simulink library "lib_controls"  (Simulink 7.9)
settings: Solver=ode45  SolverMode=SingleTasking  StartTime=0.0  StopTime=10.0  RelTol=1e-3
undefined symbols (not defined in the file or in its folder): amb_tmp, cs_charge_deplete_bool, cs_charge_pwr, cs_charge_trq, cs_clt_tmp, cs_decel_fc_off, cs_decel_regen_threshold, cs_dl_assist_trq_threshold, cs_dl_regen_trq_threshold, cs_electric_decel_spd, cs_electric_launch_spd, cs_electric_launch_spd_hi, cs_electric_launch_spd_lo, cs_eng_min_spd, cs_eng_on_soc, cs_fc_init_state, cs_fc_max_pwr_frac, cs_fc_min_pwr_frac, cs_fc_on, cs_fc_pwr_opt, cs_fc_spd_opt, cs_fuzzy_fuel_mode, cs_hi_soc, cs_hi_trq_frac, cs_lo_soc, cs_lo_trq_frac, cs_max_gc_spd, cs_max_pwr, cs_max_pwr_fall_rate, cs_max_pwr_rise_rate, cs_mc_assist_max_frac, cs_mc_assist_min_frac, cs_mc_assist_slope, cs_mc_regen_max_frac, cs_mc_regen_min_frac, cs_mc_regen_slope, cs_mean_eff, cs_mean_eff_bool, cs_min_gc_spd, cs_min_off_time, cs_min_pwr, cs_min_trq_frac, cs_mph_avg_time, cs_off_trq_frac, cs_plot_output, cs_pwr, cs_regen_avg_time, cs_scale_factor, cs_shutoff, cs_soc_range, cs_spd, cs_target_soc, cs_trq_to_soc_factor, cvt_locus_pwr, cvt_locus_spd, cyc_mph, enable_sim_stop_distance, enable_sim_stop_max_spd, enable_sim_stop_speed, enable_sim_stop_time ... (+110)
libraries: lib_controls x124, simulink3 x13, simulink x5, lib_etc x1
(part 15 of 17)

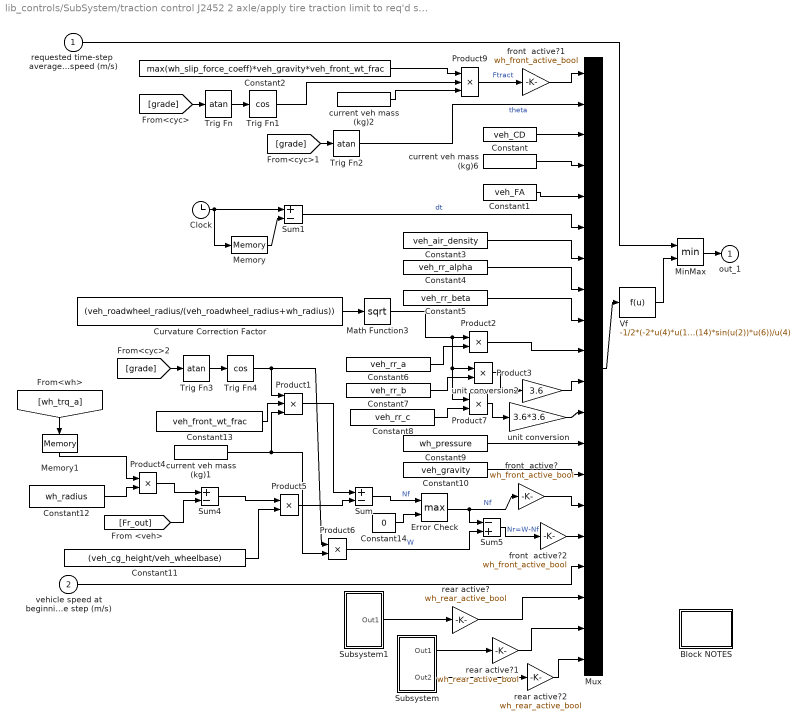
== system lib_controls/SubSystem/traction control J2452 2 axle/apply tire traction limit to req'd speed (m/s) ==
  "requested time-step  average vehicle speed (m/s) " : Inport
  vehicle speed at beginning of time step (m/s) : Inport  Port=2
  Block NOTES : Subsystem
      mask Display: disp('Block\nNOTES')
  Clock : Clock
  Constant : Constant  Value=veh_CD
  Constant1 : Constant  Value=veh_FA
  Constant10 : Constant  Value=veh_gravity
  Constant11 : Constant  Value=(veh_cg_height/veh_wheelbase)
  Constant12 : Constant  Value=wh_radius
  Constant13 : Constant  Value=veh_front_wt_frac
  Constant14 : Constant  Value=0
  Constant2 : Constant  Value=max(wh_slip_force_coeff)*veh_gravity*veh_front_wt_frac
  Constant3 : Constant  Value=veh_air_density
  Constant4 : Constant  Value=veh_rr_alpha
  Constant5 : Constant  Value=veh_rr_beta
  Constant6 : Constant  Value=veh_rr_a
  Constant7 : Constant  Value=veh_rr_b
  Constant8 : Constant  Value=veh_rr_c
  Constant9 : Constant  Value=wh_pressure
  Curvature Correction Factor : Constant  Value=(veh_roadwheel_radius/(veh_roadwheel_radius+wh_radius))  VectorParams1D=off
  Error Check : MinMax  Function=max  Inputs=2  SaturateOnIntegerOverflow=on  InputSameDT=on
  Math Function3 : Math  Operator=sqrt  SaturateOnIntegerOverflow=on
  Memory : Memory  X0=-0.1
  Memory1 : Memory  X0=-0.1
  MinMax : MinMax  Inputs=2  SaturateOnIntegerOverflow=on  InputSameDT=on
  Mux : Mux  Inputs=20
  Product1 : Product  Inputs=3  SaturateOnIntegerOverflow=on  RndMeth=Zero  InputSameDT=on  OutDataTypeStr=Inherit: Same as first input
  Product{2..7} (6 alike) : Product  SaturateOnIntegerOverflow=on  RndMeth=Zero  InputSameDT=on  OutDataTypeStr=Inherit: Same as first input
  Product9 : Product  Inputs=3  SaturateOnIntegerOverflow=on  RndMeth=Zero  InputSameDT=on  OutDataTypeStr=Inherit: Same as first input
  Subsystem : Subsystem
  Subsystem1 : Subsystem
  Sum : Sum  Inputs=+-  SaturateOnIntegerOverflow=on  InputSameDT=on  OutDataTypeStr=Inherit: Same as first input
  Sum1 : Sum  Inputs=+-  SaturateOnIntegerOverflow=on  InputSameDT=on  OutDataTypeStr=Inherit: Same as first input
  Sum4 : Sum  Inputs=+-  SaturateOnIntegerOverflow=on  InputSameDT=on  OutDataTypeStr=Inherit: Same as first input
  Sum5 : Sum  Inputs=-+  SaturateOnIntegerOverflow=on  InputSameDT=on  OutDataTypeStr=Inherit: Same as first input
  Trig Fn : Trigonometry  Operator=atan
  Trig Fn1 : Trigonometry  Operator=cos
  Trig Fn2 : Trigonometry  Operator=atan
  Trig Fn3 : Trigonometry  Operator=atan
  Trig Fn4 : Trigonometry  Operator=cos
  Vf : Fcn  Expr=-1/2*(-2*u(4)*u(17)-2*u(1)*u(6)-2*u(18)*u(6)+4*u(13)^u(8)*u(6)*(1/2*u(15))^u(9)*u(10)+4*u(13)^u(8)*u(6)*(1/2*u(19))^u(9)*u(10)+4*u(13)^u(8)*u(6)*(1/2*u(15))^u(9)*u(11)*u(17)+4*u(13)^u(8)*u(6)*(1/2*u(19))^u(9)*u(11)*u(17)+4*u(13)^u(8)*u(6)*(1/2*u(15))^u(9)*u(12)*u(17)^2+4*u(13)^u(8)*u(6)*(1/2*u(19))^u(9)*u(12)*u(17)^2+4*u(13)^u(8)*u(6)*(1/2*u(16))^u(9)*u(10)+4*u(13)^u(8)*u(6)*(1/2*u(20))^u(9)*u(10)+4*u(13)^u(8)*u(6)*(1/2*u(16))^u(9)*u(11)*u(17)+4*u(13)^u(8)*u(6)*(1/2*u(20))^u(9)*u(11)*u(17)+4*u(13)^u(8)*u(6)*(1/2*u(16))^u(9)*u(12)*u(17)^2+4*u(13)^u(8)*u(6)*(1/2*u(20))^u(9)*u(12)*u(17)^2+u(7)*u(3)*u(5)*u(17)^2*u(6)+2*u(4)*u(14)*sin(u(2))*u(6))/u(4)
  current veh mass (kg)1 : lib_controls/SubSystem/current veh mass (kg)
      settings: RTWFcnNameOpts=Auto  RTWFileNameOpts=Auto
  current veh mass (kg)2 : lib_controls/SubSystem/current veh mass (kg)
      settings: RTWFcnNameOpts=Auto  RTWFileNameOpts=Auto
  current veh mass (kg)6 : lib_controls/SubSystem/current veh mass (kg)
      settings: RTWFcnNameOpts=Auto  RTWFileNameOpts=Auto
  front  active? : Gain  Gain=wh_front_active_bool  SaturateOnIntegerOverflow=on  OutDataTypeStr=Inherit: Same as input  ParamDataTypeStr=Inherit: Same as input
  front  active?1 : Gain  Gain=wh_front_active_bool  SaturateOnIntegerOverflow=on  OutDataTypeStr=Inherit: Same as input  ParamDataTypeStr=Inherit: Same as input
  front  active?2 : Gain  Gain=wh_front_active_bool  SaturateOnIntegerOverflow=on  OutDataTypeStr=Inherit: Same as input  ParamDataTypeStr=Inherit: Same as input
  rear active? : Gain  Gain=wh_rear_active_bool  SaturateOnIntegerOverflow=on  OutDataTypeStr=Inherit: Same as input  ParamDataTypeStr=Inherit: Same as input
  rear active?1 : Gain  Gain=wh_rear_active_bool  SaturateOnIntegerOverflow=on  OutDataTypeStr=Inherit: Same as input  ParamDataTypeStr=Inherit: Same as input
  rear active?2 : Gain  Gain=wh_rear_active_bool  SaturateOnIntegerOverflow=on  OutDataTypeStr=Inherit: Same as input  ParamDataTypeStr=Inherit: Same as input
  unit conversion : Gain  Gain=3.6*3.6  SaturateOnIntegerOverflow=on  OutDataTypeStr=Inherit: Same as input  ParamDataTypeStr=Inherit: Same as input
  unit conversion2 : Gain  Gain=3.6  SaturateOnIntegerOverflow=on  OutDataTypeStr=Inherit: Same as input  ParamDataTypeStr=Inherit: Same as input
  out_1 : Outport  InitialOutput=0
  wires:
  Product7/1 -> unit conversion/1
  Constant8/1 -> Product7/2
  Product3/1 -> unit conversion2/1
  Constant7/1 -> Product3/2
  Product2/1 -> Mux/10
  Constant6/1 -> Product2/2
  Math Function3/1 -> Product7/1, Product3/1, Product2/1
  Curvature Correction Factor/1 -> Math Function3/1
  unit conversion/1 -> Mux/12
  unit conversion2/1 -> Mux/11
  Error Check/1 -> Sum5/1, front  active?/1  "Nf"
  Constant14/1 -> Error Check/2
  Sum/1 -> Error Check/1  "Nf"
  Sum5/1 -> front  active?2/1  "Nr=W-Nf"
  Product6/1 -> Sum5/2  "W"
  Memory1/1 -> Product4/1
  [wh_trq_a] -> Memory1/1
  vehicle speed at beginning of time step (m/s)/1 -> Mux/17
  current veh mass (kg)1/1 -> Product6/2, Product1/3
  Constant13/1 -> Product1/2
  Trig Fn4/1 -> Product6/1, Product1/1
  Trig Fn3/1 -> Trig Fn4/1
  [grade] -> Trig Fn3/1
  Constant10/1 -> Mux/14
  Constant9/1 -> Mux/13
  Constant5/1 -> Mux/9
  Constant4/1 -> Mux/8
  Constant3/1 -> Mux/7
  Constant1/1 -> Mux/5
  current veh mass (kg)6/1 -> Mux/4
  Constant/1 -> Mux/3
  Mux/1 -> Vf/1
  Trig Fn1/1 -> Product9/2
  current veh mass (kg)2/1 -> Product9/3
  "requested time-step  average vehicle speed (m/s) "/1 -> MinMax/1
  Constant2/1 -> Product9/1
  Trig Fn/1 -> Trig Fn1/1
  [grade] -> Trig Fn/1
  Product9/1 -> front  active?1/1  "Ftract"
  Sum1/1 -> Mux/6  "dt"
  Clock/1 -> Memory/1, Sum1/1
  Memory/1 -> Sum1/2
  [grade] -> Trig Fn2/1
  Trig Fn2/1 -> Mux/2  "theta"
  Product1/1 -> Sum/1
  MinMax/1 -> out_1/1
  Constant12/1 -> Product4/2
  Product4/1 -> Sum4/1
  [Fr_out] -> Sum4/2
  Sum4/1 -> Product5/1
  Constant11/1 -> Product5/2
  Product5/1 -> Sum/2
  Vf/1 -> MinMax/2
  Subsystem1/1(Out1) -> rear active?/1
  Subsystem/1(Out1) -> rear active?1/1
  Subsystem/2(Out2) -> rear active?2/1
  front  active?1/1 -> Mux/1
  front  active?/1 -> Mux/15
  front  active?2/1 -> Mux/16
  rear active?/1 -> Mux/18
  rear active?2/1 -> Mux/20
  rear active?1/1 -> Mux/19

== system lib_controls/electric assist control strategy bal <cs>/SOC corrected  trq req'd (N*m)/SOC  Correction  Factor ==
  note: Depending in the location of the manual
      | switches the correction factor will either
      | be a linear, quad, or cubic function within the
      | specified range
  SOC : Inport
  high soc : Inport  Port=2
  low soc : Inport  Port=3
  0.5*range : Gain  Gain=0.5  SaturateOnIntegerOverflow=on  OutDataTypeStr=Inherit: Same as input  ParamDataTypeStr=Inherit: Same as input
  Constant3 : Constant  Value=3
  Constant4 : Constant  Value=2
  Manual  Switch1 : simulink3/Nonlinear/Manual Switch  sw=0  action=0
  Manual Switch : simulink3/Nonlinear/Manual Switch  sw=1  action=0
  Math Function : Math  Operator=pow  SaturateOnIntegerOverflow=on
  Math Function1 : Math  Operator=pow  SaturateOnIntegerOverflow=on
  Multiplier6 : Product  Inputs=*/  SaturateOnIntegerOverflow=on  RndMeth=Zero  InputSameDT=on  OutDataTypeStr=Inherit: Same as first input
  Multiplier7 : Product  SaturateOnIntegerOverflow=on  RndMeth=Zero  InputSameDT=on  OutDataTypeStr=Inherit: Same as first input
  Sign : Signum
  Sum11 : Sum  Inputs=-+  SaturateOnIntegerOverflow=on  InputSameDT=on  OutDataTypeStr=Inherit: Same as first input
  Sum12 : Sum  SaturateOnIntegerOverflow=on  InputSameDT=on  OutDataTypeStr=Inherit: Same as first input
  Sum14 : Sum  Inputs=+-  SaturateOnIntegerOverflow=on  InputSameDT=on  OutDataTypeStr=Inherit: Same as first input
  mean : Gain  Gain=0.5  SaturateOnIntegerOverflow=on  OutDataTypeStr=Inherit: Same as input  ParamDataTypeStr=Inherit: Same as input
  SOC  correction  factor : Outport  InitialOutput=0
  wires:
  Multiplier7/1 -> Manual  Switch1/2
  Sign/1 -> Multiplier7/1
  Math Function1/1 -> Multiplier7/2
  Manual  Switch1/1 -> SOC  correction  factor/1
  Manual Switch/1 -> Manual  Switch1/1
  Multiplier6/1 -> Math Function1/1, Sign/1, Manual Switch/1, Math Function/1
  Constant4/1 -> Math Function1/2
  Math Function/1 -> Manual Switch/2
  Constant3/1 -> Math Function/2
  0.5*range/1 -> Multiplier6/2
  Sum11/1 -> Multiplier6/1
  low soc/1 -> Sum14/2, Sum12/2
  high soc/1 -> Sum14/1, Sum12/1
  Sum14/1 -> 0.5*range/1
  Sum12/1 -> mean/1
  mean/1 -> Sum11/2
  SOC/1 -> Sum11/1

== system lib_controls/electric assist control strategy bal <cs>/SOC corrected  trq req'd (N*m)/max trq  and  trq frac ==
  trq req : Inport
  spd req : Inport  Port=2
  Constant : Constant  Value=eps
  Multiplier3 : Product  Inputs=*/  SaturateOnIntegerOverflow=on  RndMeth=Zero  InputSameDT=on  OutDataTypeStr=Inherit: Same as first input
  Saturation4 : Saturate  UpperLimit=inf  LowerLimit=0
  Saturation7 : Saturate  UpperLimit=1  LowerLimit=0
  Sum8 : Sum  Inputs=2  SaturateOnIntegerOverflow=on  InputSameDT=on  OutDataTypeStr=Inherit: Same as first input
  max_torque  lookup : Lookup  InputValues=fc_map_spd*fc_spd_scale  Table=fc_max_trq*fc_trq_scale  SaturateOnIntegerOverflow=on
  max trq : Outport  InitialOutput=0
  trq frac : Outport  Port=2  InitialOutput=0
  wires:
  Saturation7/1 -> trq frac/1
  spd req/1 -> max_torque  lookup/1
  Saturation4/1 -> max trq/1, Sum8/1
  max_torque  lookup/1 -> Saturation4/1
  Constant/1 -> Sum8/2
  Sum8/1 -> Multiplier3/2
  Multiplier3/1 -> Saturation7/1
  trq req/1 -> Multiplier3/1

== system lib_controls/electric assist control strategy bal <cs>/SOC corrected  trq req'd (N*m)/trq  Correction  Factor ==
  note: Depending in the location of the manual
      | switches the correction factor will either
      | be a linear, quad, or cubic function within the
      | specified range
  trq : Inport
  high trq : Inport  Port=2
  low trq : Inport  Port=3
  0.5*range : Gain  Gain=0.5  SaturateOnIntegerOverflow=on  OutDataTypeStr=Inherit: Same as input  ParamDataTypeStr=Inherit: Same as input
  Constant3 : Constant  Value=3
  Constant4 : Constant  Value=2
  Manual Switch : simulink3/Nonlinear/Manual Switch  sw=1  action=0
  Manual Switch1 : simulink3/Nonlinear/Manual Switch  sw=0  action=0
  Math Function : Math  Operator=pow  SaturateOnIntegerOverflow=on
  Math Function1 : Math  Operator=pow  SaturateOnIntegerOverflow=on
  Multiplier6 : Product  Inputs=*/  SaturateOnIntegerOverflow=on  RndMeth=Zero  InputSameDT=on  OutDataTypeStr=Inherit: Same as first input
  Multiplier7 : Product  SaturateOnIntegerOverflow=on  RndMeth=Zero  InputSameDT=on  OutDataTypeStr=Inherit: Same as first input
  Sign : Signum
  Sum11 : Sum  Inputs=-+  SaturateOnIntegerOverflow=on  InputSameDT=on  OutDataTypeStr=Inherit: Same as first input
  Sum12 : Sum  SaturateOnIntegerOverflow=on  InputSameDT=on  OutDataTypeStr=Inherit: Same as first input
  Sum14 : Sum  Inputs=+-  SaturateOnIntegerOverflow=on  InputSameDT=on  OutDataTypeStr=Inherit: Same as first input
  mean : Gain  Gain=0.5  SaturateOnIntegerOverflow=on  OutDataTypeStr=Inherit: Same as input  ParamDataTypeStr=Inherit: Same as input
  trq  correction  factor : Outport  InitialOutput=0
  wires:
  Multiplier7/1 -> Manual Switch1/2
  Sign/1 -> Multiplier7/1
  Math Function1/1 -> Multiplier7/2
  Manual Switch1/1 -> trq  correction  factor/1
  Manual Switch/1 -> Manual Switch1/1
  Multiplier6/1 -> Math Function1/1, Sign/1, Manual Switch/1, Math Function/1
  Constant4/1 -> Math Function1/2
  Math Function/1 -> Manual Switch/2
  Constant3/1 -> Math Function/2
  0.5*range/1 -> Multiplier6/2
  Sum11/1 -> Multiplier6/1
  low trq/1 -> Sum14/2, Sum12/2
  high trq/1 -> Sum14/1, Sum12/1
  Sum14/1 -> 0.5*range/1
  Sum12/1 -> mean/1
  mean/1 -> Sum11/2
  trq/1 -> Sum11/1

== system lib_controls/electric assist control strategy  CVT <cs>/FC trq and spd/Block NOTES ==
  note: In modes 1 and 2 engine is off and trq req is zero
      | In mode 3 a charge pwr is added to the pwr req and the spd
      | and trq are then determined based on modified pwr
      | In Mode 4 the trq is determined by fc IOL

== system lib_controls/electric assist control strategy  CVT <cs>/FC trq and spd/Speed Interp ==
  Mode : Inport
  pwr req : Inport  Port=2
  Multiport Switch : MultiPortSwitch  Inputs=4  zeroidx=off  SaturateOnIntegerOverflow=on  InputSameDT=on
  Saturation3 : Saturate  UpperLimit=max(ptc_fc_mc_iol_pwr_vec)  LowerLimit=min(ptc_fc_mc_iol_pwr_vec)
  Saturation6 : Saturate  UpperLimit=max(ptc_mc_iol_pwr_vec)  LowerLimit=min(ptc_mc_iol_pwr_vec)
  Saturation7 : Saturate  UpperLimit=max(ptc_fc_iol_pwr_vec)  LowerLimit=min(ptc_fc_iol_pwr_vec)
  Saturation8 : Saturate  UpperLimit=max(ptc_mc_gen_iol_pwr_vec)  LowerLimit=min(ptc_mc_gen_iol_pwr_vec)
  desired engine spd engine and motor : Lookup  InputValues=ptc_fc_mc_iol_pwr_vec  Table=ptc_fc_mc_iol_spd_vec  SaturateOnIntegerOverflow=on
  desired engine spd engine only : Lookup  InputValues=ptc_fc_iol_pwr_vec  Table=ptc_fc_iol_spd_vec  SaturateOnIntegerOverflow=on
  desired motor spd motor only : Lookup  InputValues=ptc_mc_iol_pwr_vec  Table=ptc_mc_iol_spd_vec  SaturateOnIntegerOverflow=on
  desired motor spd motor only regen : Lookup  InputValues=fliplr(ptc_mc_gen_iol_pwr_vec)  Table=fliplr(ptc_mc_gen_iol_spd_vec)  SaturateOnIntegerOverflow=on
  input spd : Outport
  wires:
  Saturation6/1 -> desired motor spd motor only/1
  Saturation8/1 -> desired motor spd motor only regen/1
  Saturation7/1 -> desired engine spd engine only/1
  Saturation3/1 -> desired engine spd engine and motor/1
  Multiport Switch/1 -> input spd/1
  Mode/1 -> Multiport Switch/1
  pwr req/1 -> Saturation3/1, Saturation7/1, Saturation6/1, Saturation8/1
  desired motor spd motor only regen/1 -> Multiport Switch/2
  desired motor spd motor only/1 -> Multiport Switch/3
  desired engine spd engine only/1 -> Multiport Switch/4
  desired engine spd engine and motor/1 -> Multiport Switch/5

== system lib_controls/electric assist control strategy  CVT <cs>/FC trq and spd/chg pwr req'd (W) ==
  Constant : Constant  Value=cs_charge_pwr*fc_trq_scale
  Goal : Constant  Value=(cs_lo_soc+cs_hi_soc)/2
  Product : Product  SaturateOnIntegerOverflow=on  RndMeth=Zero  InputSameDT=on  OutDataTypeStr=Inherit: Same as first input
  Product1 : Product  Inputs=*/  SaturateOnIntegerOverflow=on  RndMeth=Zero  InputSameDT=on  OutDataTypeStr=Inherit: Same as first input
  Range : Constant  Value=(cs_hi_soc-cs_lo_soc)/2
  Saturation : Saturate  UpperLimit=inf  LowerLimit=-inf
  Sum : Sum  Inputs=-+  SaturateOnIntegerOverflow=on  InputSameDT=on  OutDataTypeStr=Inherit: Same as first input
  add'l pwr req'd (W) : Outport
  wires:
  [SOC] -> Sum/1
  Goal/1 -> Sum/2
  Range/1 -> Product1/2
  Sum/1 -> Product1/1
  Product1/1 -> Product/2
  Constant/1 -> Product/1
  Product/1 -> Saturation/1
  Saturation/1 -> add'l pwr req'd (W)/1

== system lib_controls/electric assist control strategy  CVT <cs>/FC trq and spd/old engine spin up ==
  In1 : Inport
  In2 : Inport  Port=2
  Constant6 : Constant  Value=0
  Constant7 : Constant  Value=eps
  Gain : Gain  Gain=.5  SaturateOnIntegerOverflow=on  OutDataTypeStr=Inherit: Same as input  ParamDataTypeStr=Inherit: Same as input
  Logical Operator : Logic
  Logical Operator1 : Logic  Operator=NOT  Inputs=1
  Memory : Memory
  Relational Operator : RelationalOperator  Operator=>  InputSameDT=on
  Switch2 : Switch  Threshold=eps  SaturateOnIntegerOverflow=on  InputSameDT=on
  Switch3 : Switch  Threshold=eps  SaturateOnIntegerOverflow=on  InputSameDT=on
  Terminator : Terminator
  wires:
  In2/1 -> Switch2/2
  Switch3/1 -> Terminator/1
  Constant6/1 -> Switch2/3
  Logical Operator/1 -> Switch3/2
  Constant7/1 -> Relational Operator/2
  Memory/1 -> Logical Operator1/1
  Relational Operator/1 -> Logical Operator/1, Memory/1
  Logical Operator1/1 -> Logical Operator/2
  Switch2/1 -> Relational Operator/1, Gain/1, Switch3/3
  Gain/1 -> Switch3/1
  In1/1 -> Switch2/1

== system lib_controls/fuel cell adaptive <cs>/Delta SOC expected from regen/Subsystem ==
  in_1 : Inport
  1/average time : Constant  Value=1/n
  Integrator : Integrator
  Product : Product  SaturateOnIntegerOverflow=on  RndMeth=Zero  InputSameDT=on  OutDataTypeStr=Inherit: Same as first input
  Sum : Sum  Inputs=+-  SaturateOnIntegerOverflow=on  InputSameDT=on  OutDataTypeStr=Inherit: Same as first input
  Transport Delay : TransportDelay  DelayTime=n
  out_1 : Outport  InitialOutput=0
  wires:
  1/average time/1 -> Product/2
  Product/1 -> out_1/1
  in_1/1 -> Integrator/1
  Sum/1 -> Product/1
  Transport Delay/1 -> Sum/2
  Integrator/1 -> Transport Delay/1, Sum/1

== system lib_controls/fuel cell control strategy <cs>/FC on/Subsystem ==
  in_1 : Inport
  Constant1 : Constant  Value=n
  Integrator : Integrator
  Product : Product  Inputs=*/  SaturateOnIntegerOverflow=on  RndMeth=Zero  InputSameDT=on  OutDataTypeStr=Inherit: Same as first input
  Sum : Sum  Inputs=+-  SaturateOnIntegerOverflow=on  InputSameDT=on  OutDataTypeStr=Inherit: Same as first input
  Transport Delay : TransportDelay  DelayTime=n
  out_1 : Outport  InitialOutput=0
  wires:
  Constant1/1 -> Product/2
  Product/1 -> out_1/1
  in_1/1 -> Integrator/1
  Sum/1 -> Product/1
  Transport Delay/1 -> Sum/2
  Integrator/1 -> Transport Delay/1, Sum/1

== system lib_controls/fuel cell control strategy <cs>/FC on/dt ==
  Clock : Clock
  Memory1 : Memory  X0=-1
  Sum1 : Sum  Inputs=+-  SaturateOnIntegerOverflow=on  InputSameDT=on  OutDataTypeStr=Inherit: Same as first input
  out_1 : Outport  InitialOutput=0
  wires:
  Sum1/1 -> out_1/1
  Memory1/1 -> Sum1/2
  Clock/1 -> Memory1/1, Sum1/1

== system lib_controls/fuel cell control strategy <cs>/FC on/just shut  down ==
  state : Inport
  Logical Operator : Logic
  Logical Operator1 : Logic  Operator=NOT  Inputs=1
  Memory1 : Memory  X0=1
  trigger : Outport  InitialOutput=0
  wires:
  Logical Operator/1 -> trigger/1
  Memory1/1 -> Logical Operator/2
  state/1 -> Memory1/1, Logical Operator1/1
  Logical Operator1/1 -> Logical Operator/1

== system lib_controls/fuel cell control strategy <cs>/FC on/no-lag Reset Integrator ==
  in_1 : Inport
  in_2 : Inport  Port=2
  in_3 : Inport  Port=3
  Constant : Constant  Value=0
  Memory : Memory  X0=initval
  Product : Product  SaturateOnIntegerOverflow=on  RndMeth=Zero  InputSameDT=on  OutDataTypeStr=Inherit: Same as first input
  Sum : Sum  SaturateOnIntegerOverflow=on  InputSameDT=on  OutDataTypeStr=Inherit: Same as first input
  Switch : Switch  Threshold=eps  SaturateOnIntegerOverflow=on  InputSameDT=on
  dt : Subsystem
  in_2==0 : RelationalOperator  Operator===  InputSameDT=on
  out_1 : Outport  InitialOutput=0
  wires:
  Constant/1 -> in_2==0/2
  in_2==0/1 -> Switch/2
  Switch/1 -> Memory/1, out_1/1
  Sum/1 -> Switch/1
  Memory/1 -> Sum/1
  Product/1 -> Sum/2
  dt/1(out_1) -> Product/1
  in_1/1 -> Product/2
  in_2/1 -> in_2==0/1
  in_3/1 -> Switch/3

== system lib_controls/fuel cell control strategy <cs>/FC pwr command, modified by SOC/Block NOTES ==
  note: 1/5/98/98:tm  Modified calculation of additional power required to maintain goal SOC
      | (SOC_goal - SOC_actual) / (0.5*SOC_range) * cs_charge_pwr
      | therefore when
      | actual_SOC=cs_lo_soc ==> 1.0  *cs_charge_pwr
      | actual_SOC=goal_SOC ==> 0.0  *cs_charge_pwr
      | actual_SOC=cs_hi_soc ==> -1.0 * cs_charge_pwr
  note: This block determines the additional power required of the fuel convertor
      |  to maintian an SOC equal to the average of cs_hi_soc and cs_lo_soc.

== system lib_controls/series hybrid control stategy  <cs>/FC on/Subsystem ==
  in_1 : Inport
  Constant1 : Constant  Value=n
  Integrator : Integrator
  Product : Product  Inputs=*/  SaturateOnIntegerOverflow=on  RndMeth=Zero  InputSameDT=on  OutDataTypeStr=Inherit: Same as first input
  Sum : Sum  Inputs=+-  SaturateOnIntegerOverflow=on  InputSameDT=on  OutDataTypeStr=Inherit: Same as first input
  Transport Delay : TransportDelay  DelayTime=n
  out_1 : Outport  InitialOutput=0
  wires:
  Integrator/1 -> Sum/1, Transport Delay/1
  Transport Delay/1 -> Sum/2
  Sum/1 -> Product/1
  in_1/1 -> Integrator/1
  Product/1 -> out_1/1
  Constant1/1 -> Product/2

== system lib_controls/series hybrid control stategy  <cs>/FC on/dt ==
  Clock : Clock
  Memory1 : Memory  X0=-1
  Sum1 : Sum  Inputs=+-  SaturateOnIntegerOverflow=on  InputSameDT=on  OutDataTypeStr=Inherit: Same as first input
  out_1 : Outport  InitialOutput=0
  wires:
  Clock/1 -> Sum1/1, Memory1/1
  Memory1/1 -> Sum1/2
  Sum1/1 -> out_1/1

== system lib_controls/series hybrid control stategy  <cs>/FC on/just shut  down ==
  state : Inport
  Logical Operator : Logic
  Logical Operator1 : Logic  Operator=NOT  Inputs=1
  Memory1 : Memory  X0=1
  trigger : Outport  InitialOutput=0
  wires:
  Logical Operator1/1 -> Logical Operator/1
  state/1 -> Logical Operator1/1, Memory1/1
  Memory1/1 -> Logical Operator/2
  Logical Operator/1 -> trigger/1

== system lib_controls/series hybrid control stategy  <cs>/FC on/no-lag Reset Integrator ==
  in_1 : Inport
  in_2 : Inport  Port=2
  in_3 : Inport  Port=3
  Constant : Constant  Value=0
  Memory : Memory  X0=initval
  Product : Product  SaturateOnIntegerOverflow=on  RndMeth=Zero  InputSameDT=on  OutDataTypeStr=Inherit: Same as first input
  Sum : Sum  SaturateOnIntegerOverflow=on  InputSameDT=on  OutDataTypeStr=Inherit: Same as first input
  Switch : Switch  Threshold=eps  SaturateOnIntegerOverflow=on  InputSameDT=on
  dt : Subsystem
  in_2==0 : RelationalOperator  Operator===  InputSameDT=on
  out_1 : Outport  InitialOutput=0
  wires:
  in_3/1 -> Switch/3
  in_2/1 -> in_2==0/1
  in_1/1 -> Product/2
  dt/1(out_1) -> Product/1
  Product/1 -> Sum/2
  Memory/1 -> Sum/1
  Sum/1 -> Switch/1
  Switch/1 -> out_1/1, Memory/1
  in_2==0/1 -> Switch/2
  Constant/1 -> in_2==0/2

== system lib_controls/series hybrid control stategy  <cs>/FC pwr command, modified by SOC/Block NOTES ==
  note: This block determines the additional power required of the fuel convertor
      |  to maintian an SOC equal to the average of cs_hi_soc and cs_lo_soc.
  note: 1/5/98/98:tm  Modified calculation of additional power required to maintain goal SOC
      | (SOC_goal - SOC_actual) / (0.5*SOC_range) * cs_charge_pwr
      | therefore when
      | actual_SOC=cs_lo_soc ==> 1.0  *cs_charge_pwr
      | actual_SOC=goal_SOC ==> 0.0  *cs_charge_pwr
      | actual_SOC=cs_hi_soc ==> -1.0 * cs_charge_pwr
      |
      | 2/6/01:tm added if battery disabled - do not modify request

== system lib_controls/series hybrid control stategy  <cs>/FC trq and spd/Block NOTES ==
  note: This block determines the required fuel converter torque and speed from the
      | required power using a vector usually representing the locus of best efficiency
      | or lowest emissions points in the map.  The speed request is cut in half if it is
      | nonzero and preceded by a zero speed request to account for the fact that all
      | ADVISOR's drivetrain components deal in speeds averaged over the time step.
      | A speed command here of 1/2 of max. engine speed means that the AVERAGE
      | engine speed required is 1/2 of max.  If the previous speed was zero, that means
      | that the speed at the end of the current time step must be equal to max. engine
      | speed.

== system lib_controls/<vc> conv/clutch control/gearbox speed estimator/Block NOTES ==
  note: The requested engine speed is replaced by an estimate of the
      | engine's previous speed whenever the vehicle missed the trace
      |  by more than 1 mph on the last time step.

== system lib_controls/<vc> conv/clutch control/gearbox speed estimator/dt ==
  Clock : Clock
  Memory1 : Memory  X0=-1
  Sum4 : Sum  Inputs=+-  SaturateOnIntegerOverflow=on  InputSameDT=on  OutDataTypeStr=Inherit: Same as first input
  Out1 : Outport  InitialOutput=0
  wires:
  Clock/1 -> Sum4/1, Memory1/1
  Memory1/1 -> Sum4/2
  Sum4/1 -> Out1/1

== system lib_controls/<vc> conv/gearbox  control/downshift  command/load fraction ==
  In1 : Inport
  S-Function : S-Function  FunctionName=sfun_gearbox  Parameters=load, spd  EnableBusSupport=off
  Out1 : Outport  InitialOutput=0
  wires:
  S-Function/1 -> Out1/1
  In1/1 -> S-Function/1

== system lib_controls/<vc> conv/gearbox  control/gearbox speed estimator/Block NOTES ==
  note: The requested engine speed is replaced by an estimate of the
      | engine's previous speed whenever the vehicle missed the trace
      |  by more than 1 mph on the last time step.

== system lib_controls/<vc> conv/gearbox  control/gearbox speed estimator/dt ==
  Clock : Clock
  Memory1 : Memory  X0=-1
  Sum4 : Sum  Inputs=+-  SaturateOnIntegerOverflow=on  InputSameDT=on  OutDataTypeStr=Inherit: Same as first input
  Out1 : Outport  InitialOutput=0
  wires:
  Clock/1 -> Sum4/1, Memory1/1
  Memory1/1 -> Sum4/2
  Sum4/1 -> Out1/1

== system lib_controls/<vc> conv/gearbox  control/shifting1/time since last shift ==
  in_1 : Inport
  just shifted : Subsystem
      mask Display: disp('just\nshifted')
  timer : Subsystem
      mask Display: disp('timer')
  out_1 : Outport  InitialOutput=0
  wires:
  timer/1(time) -> out_1/1
  just shifted/1(out_1) -> timer/1(trigger)
  in_1/1 -> just shifted/1(in_1)

== system lib_controls/<vc> conv/gearbox  control/upshift  command/load fraction ==
  In1 : Inport
  S-Function : S-Function  FunctionName=sfun_gearbox  Parameters=load, spd  EnableBusSupport=off
  Out1 : Outport  InitialOutput=0
  wires:
  S-Function/1 -> Out1/1
  In1/1 -> S-Function/1

== system lib_controls/<vc> conv Saber custom/clutch control/gearbox speed estimator/Block NOTES ==
  note: The requested engine speed is replaced by an estimate of the
      | engine's previous speed whenever the vehicle missed the trace
      |  by more than 1 mph on the last time step.

== system lib_controls/<vc> conv Saber custom/clutch control/gearbox speed estimator/dt ==
  Clock : Clock
  Memory1 : Memory  X0=-1
  Sum4 : Sum  Inputs=+-  SaturateOnIntegerOverflow=on  InputSameDT=on  OutDataTypeStr=Inherit: Same as first input
  Out1 : Outport  InitialOutput=0
  wires:
  Sum4/1 -> Out1/1
  Memory1/1 -> Sum4/2
  Clock/1 -> Memory1/1, Sum4/1

== system lib_controls/<vc> conv Saber custom/gearbox  control/downshift  command/load fraction ==
  In1 : Inport
  S-Function : S-Function  FunctionName=sfun_gearbox  Parameters=load, spd  EnableBusSupport=off
  Out1 : Outport  InitialOutput=0
  wires:
  In1/1 -> S-Function/1
  S-Function/1 -> Out1/1

== system lib_controls/<vc> conv Saber custom/gearbox  control/gearbox speed estimator/Block NOTES ==
  note: The requested engine speed is replaced by an estimate of the
      | engine's previous speed whenever the vehicle missed the trace
      |  by more than 1 mph on the last time step.

== system lib_controls/<vc> conv Saber custom/gearbox  control/gearbox speed estimator/dt ==
  Clock : Clock
  Memory1 : Memory  X0=-1
  Sum4 : Sum  Inputs=+-  SaturateOnIntegerOverflow=on  InputSameDT=on  OutDataTypeStr=Inherit: Same as first input
  Out1 : Outport  InitialOutput=0
  wires:
  Sum4/1 -> Out1/1
  Memory1/1 -> Sum4/2
  Clock/1 -> Memory1/1, Sum4/1

== system lib_controls/<vc> conv Saber custom/gearbox  control/shifting1/time since last shift ==
  in_1 : Inport
  just shifted : Subsystem
      mask Display: disp('just\nshifted')
  timer : Subsystem
      mask Display: disp('timer')
  out_1 : Outport  InitialOutput=0
  wires:
  in_1/1 -> just shifted/1(in_1)
  just shifted/1(out_1) -> timer/1(trigger)
  timer/1(time) -> out_1/1

== system lib_controls/<vc> conv Saber custom/gearbox  control/upshift  command/load fraction ==
  In1 : Inport
  S-Function : S-Function  FunctionName=sfun_gearbox  Parameters=load, spd  EnableBusSupport=off
  Out1 : Outport  InitialOutput=0
  wires:
  In1/1 -> S-Function/1
  S-Function/1 -> Out1/1

== system lib_controls/<vc> conv auto/gearbox control for use w/ AT/downshift  command/load fraction ==
  In1 : Inport
  S-Function : S-Function  FunctionName=sfun_gearbox  Parameters=load, spd  EnableBusSupport=off
  Out1 : Outport  InitialOutput=0
  wires:
  In1/1 -> S-Function/1
  S-Function/1 -> Out1/1

== system lib_controls/<vc> conv auto/gearbox control for use w/ AT/downshift  command1/load fraction ==
  In1 : Inport
  S-Function : S-Function  FunctionName=sfun_gearbox  Parameters=load, spd  EnableBusSupport=off
  Out1 : Outport  InitialOutput=0
  wires:
  S-Function/1 -> Out1/1
  In1/1 -> S-Function/1

== system lib_controls/<vc> conv auto/gearbox control for use w/ AT/est. engine trq and spd/Block NOTES ==
  note: Estimate engine torque and speed associated with the previous gear, assuming that
      | the gearbox efficiency is constant.

== system lib_controls/<vc> conv auto/gearbox control for use w/ AT/est. engine trq and spd/K_adv ==
  "Req'd output trq and spd (Nm), (rad/s)" : Inport
  K_adv=wout/(Tout)^0.5 : Fcn  Expr=u[2]/u[1]^0.5
  Saturation : Saturate  UpperLimit=max(htc_k_adv)  LowerLimit=min(htc_k_adv)
  Saturation2 : Saturate  UpperLimit=inf  LowerLimit=eps
  K_adv : Outport
  wires:
  Saturation/1 -> K_adv/1
  K_adv=wout/(Tout)^0.5/1 -> Saturation/1
  Saturation2/1 -> K_adv=wout/(Tout)^0.5/1
  "Req'd output trq and spd (Nm), (rad/s)"/1 -> Saturation2/1

== system lib_controls/<vc> conv auto/gearbox control for use w/ AT/est. engine trq and spd assuming lockup/Block NOTES ==
  note: Estimate engine torque and speed associated with the current gear, assuming that
      | the gearbox efficiency is constant.

== system lib_controls/<vc> conv auto/gearbox control for use w/ AT/shifting1/time since last shift ==
  in_1 : Inport
  just shifted : Subsystem
      mask Display: disp('just\nshifted')
  timer : Subsystem
      mask Display: disp('timer')
  out_1 : Outport  InitialOutput=0
  wires:
  timer/1(time) -> out_1/1
  just shifted/1(out_1) -> timer/1(trigger)
  in_1/1 -> just shifted/1(in_1)

== system lib_controls/<vc> conv auto/gearbox control for use w/ AT/upshift  command/load fraction ==
  In1 : Inport
  S-Function : S-Function  FunctionName=sfun_gearbox  Parameters=load, spd  EnableBusSupport=off
  Out1 : Outport  InitialOutput=0
  wires:
  In1/1 -> S-Function/1
  S-Function/1 -> Out1/1

== system lib_controls/<vc> conv auto Saber custom/gearbox control for use w/ AT/downshift  command/load fraction ==
  In1 : Inport
  S-Function : S-Function  FunctionName=sfun_gearbox  Parameters=load, spd  EnableBusSupport=off
  Out1 : Outport  InitialOutput=0
  wires:
  S-Function/1 -> Out1/1
  In1/1 -> S-Function/1

== system lib_controls/<vc> conv auto Saber custom/gearbox control for use w/ AT/downshift  command1/load fraction ==
  In1 : Inport
  S-Function : S-Function  FunctionName=sfun_gearbox  Parameters=load, spd  EnableBusSupport=off
  Out1 : Outport  InitialOutput=0
  wires:
  In1/1 -> S-Function/1
  S-Function/1 -> Out1/1

== system lib_controls/<vc> conv auto Saber custom/gearbox control for use w/ AT/est. engine trq and spd/Block NOTES ==
  note: Estimate engine torque and speed associated with the previous gear, assuming that
      | the gearbox efficiency is constant.

== system lib_controls/<vc> conv auto Saber custom/gearbox control for use w/ AT/est. engine trq and spd/K_adv ==
  "Req'd output trq and spd (Nm), (rad/s)" : Inport
  K_adv=wout/(Tout)^0.5 : Fcn  Expr=u[2]/u[1]^0.5
  Saturation : Saturate  UpperLimit=max(htc_k_adv)  LowerLimit=min(htc_k_adv)
  Saturation2 : Saturate  UpperLimit=inf  LowerLimit=eps
  K_adv : Outport
  wires:
  "Req'd output trq and spd (Nm), (rad/s)"/1 -> Saturation2/1
  Saturation2/1 -> K_adv=wout/(Tout)^0.5/1
  K_adv=wout/(Tout)^0.5/1 -> Saturation/1
  Saturation/1 -> K_adv/1

== system lib_controls/<vc> conv auto Saber custom/gearbox control for use w/ AT/est. engine trq and spd/accessories (Nm) ==
  Out1 : Outport
  wires:
  [fc_acc_trq_r] -> Out1/1

== system lib_controls/<vc> conv auto Saber custom/gearbox control for use w/ AT/est. engine trq and spd assuming lockup/Block NOTES ==
  note: Estimate engine torque and speed associated with the current gear, assuming that
      | the gearbox efficiency is constant.

== system lib_controls/<vc> conv auto Saber custom/gearbox control for use w/ AT/est. engine trq and spd assuming lockup/accessories (Nm) ==
  T_acc : Outport  InitialOutput=0
  wires:
  [fc_acc_trq_r] -> T_acc/1

== system lib_controls/<vc> conv auto Saber custom/gearbox control for use w/ AT/shifting1/time since last shift ==
  in_1 : Inport
  just shifted : Subsystem
      mask Display: disp('just\nshifted')
  timer : Subsystem
      mask Display: disp('timer')
  out_1 : Outport  InitialOutput=0
  wires:
  in_1/1 -> just shifted/1(in_1)
  just shifted/1(out_1) -> timer/1(trigger)
  timer/1(time) -> out_1/1

== system lib_controls/<vc> conv auto Saber custom/gearbox control for use w/ AT/upshift  command/load fraction ==
  In1 : Inport
  S-Function : S-Function  FunctionName=sfun_gearbox  Parameters=load, spd  EnableBusSupport=off
  Out1 : Outport  InitialOutput=0
  wires:
  S-Function/1 -> Out1/1
  In1/1 -> S-Function/1

== system lib_controls/<vc> ev/gearbox control for series  HV and EV/downshift  command/load fraction ==
  In1 : Inport
  S-Function : S-Function  FunctionName=sfun_gearbox  Parameters=load, spd  EnableBusSupport=off
  Out1 : Outport  InitialOutput=0
  wires:
  In1/1 -> S-Function/1
  S-Function/1 -> Out1/1

== system lib_controls/<vc> ev/gearbox control for series  HV and EV/gearbox speed estimator/Block NOTES ==
  note: The requested motor speed is replaced by an estimate of the
      | engine's previous speed whenever the vehicle missed the trace
      |  by more than 1 mph on the last time step.

== system lib_controls/<vc> ev/gearbox control for series  HV and EV/gearbox speed estimator/dt ==
  Clock : Clock
  Memory1 : Memory  X0=-1
  Sum4 : Sum  Inputs=+-  SaturateOnIntegerOverflow=on  InputSameDT=on  OutDataTypeStr=Inherit: Same as first input
  Out1 : Outport  InitialOutput=0
  wires:
  Sum4/1 -> Out1/1
  Memory1/1 -> Sum4/2
  Clock/1 -> Memory1/1, Sum4/1

== system lib_controls/<vc> ev/gearbox control for series  HV and EV/shifting1/time since last shift ==
  in_1 : Inport
  just shifted : Subsystem
      mask Display: disp('just\nshifted')
  timer : Subsystem
      mask Display: disp('timer')
  out_1 : Outport  InitialOutput=0
  wires:
  in_1/1 -> just shifted/1(in_1)
  just shifted/1(out_1) -> timer/1(trigger)
  timer/1(time) -> out_1/1

== system lib_controls/<vc> ev/gearbox control for series  HV and EV/upshift  command/load fraction ==
  In1 : Inport
  S-Function : S-Function  FunctionName=sfun_gearbox  Parameters=load, spd  EnableBusSupport=off
  Out1 : Outport  InitialOutput=0
  wires:
  In1/1 -> S-Function/1
  S-Function/1 -> Out1/1

== system lib_controls/<vc> fuel cell/gearbox control for series  HV and EV/downshift  command/load fraction ==
  In1 : Inport
  S-Function : S-Function  FunctionName=sfun_gearbox  Parameters=load, spd  EnableBusSupport=off
  Out1 : Outport  InitialOutput=0
  wires:
  In1/1 -> S-Function/1
  S-Function/1 -> Out1/1

== system lib_controls/<vc> fuel cell/gearbox control for series  HV and EV/gearbox speed estimator/Block NOTES ==
  note: The requested motor speed is replaced by an estimate of the
      | engine's previous speed whenever the vehicle missed the trace
      |  by more than 1 mph on the last time step.

== system lib_controls/<vc> fuel cell/gearbox control for series  HV and EV/gearbox speed estimator/dt ==
  Clock : Clock
  Memory1 : Memory  X0=-1
  Sum4 : Sum  Inputs=+-  SaturateOnIntegerOverflow=on  InputSameDT=on  OutDataTypeStr=Inherit: Same as first input
  Out1 : Outport  InitialOutput=0
  wires:
  Sum4/1 -> Out1/1
  Memory1/1 -> Sum4/2
  Clock/1 -> Memory1/1, Sum4/1

== system lib_controls/<vc> fuel cell/gearbox control for series  HV and EV/shifting1/time since last shift ==
  in_1 : Inport
  just shifted : Subsystem
      mask Display: disp('just\nshifted')
  timer : Subsystem
      mask Display: disp('timer')
  out_1 : Outport  InitialOutput=0
  wires:
  in_1/1 -> just shifted/1(in_1)
  just shifted/1(out_1) -> timer/1(trigger)
  timer/1(time) -> out_1/1

== system lib_controls/<vc> fuel cell/gearbox control for series  HV and EV/upshift  command/load fraction ==
  In1 : Inport
  S-Function : S-Function  FunctionName=sfun_gearbox  Parameters=load, spd  EnableBusSupport=off
  Out1 : Outport  InitialOutput=0
  wires:
  In1/1 -> S-Function/1
  S-Function/1 -> Out1/1

== system lib_controls/<vc> insight/parallel clutch control/gearbox speed estimator/Block NOTES ==
  note: The requested engine speed is replaced by an estimate of the
      | engine's previous speed whenever the vehicle missed the trace
      |  by more than 1 mph on the last time step.

== system lib_controls/<vc> insight/parallel clutch control/gearbox speed estimator/dt ==
  Clock : Clock
  Memory1 : Memory  X0=-1
  Sum4 : Sum  Inputs=+-  SaturateOnIntegerOverflow=on  InputSameDT=on  OutDataTypeStr=Inherit: Same as first input
  Out1 : Outport  InitialOutput=0
  wires:
  Sum4/1 -> Out1/1
  Memory1/1 -> Sum4/2
  Clock/1 -> Memory1/1, Sum4/1

== system lib_controls/<vc> insight/pre-TX parallel gearbox control/allow upshift?/Block NOTES1 ==
  note: This block prevents an upshift if it the engine is not on and
      | the upshift would make the motor power low enough that it
      | could not provide the required input power.  However, an upshift
      | is allowed if to stay in the current gear would put the motor
      | beyond 95% of its maximum speed.
      |
      | This block is to be used in pretransmission parallel hybrids
      | (where the engine and motor torques are combined on the
      | engine side of the transmission) ONLY.

== system lib_controls/<vc> insight/pre-TX parallel gearbox control/downshift  command/load fraction ==
  In1 : Inport
  S-Function : S-Function  FunctionName=sfun_gearbox  Parameters=load, spd  EnableBusSupport=off
  Out1 : Outport  InitialOutput=0
  wires:
  S-Function/1 -> Out1/1
  In1/1 -> S-Function/1

== system lib_controls/<vc> insight/pre-TX parallel gearbox control/gearbox speed estimator/Block NOTES ==
  note: The requested engine speed is replaced by an estimate of the
      | engine's previous speed whenever the vehicle missed the trace
      |  by more than 1 mph on the last time step.

== system lib_controls/<vc> insight/pre-TX parallel gearbox control/gearbox speed estimator/dt ==
  Clock : Clock
  Memory1 : Memory  X0=-1
  Sum4 : Sum  Inputs=+-  SaturateOnIntegerOverflow=on  InputSameDT=on  OutDataTypeStr=Inherit: Same as first input
  Out1 : Outport  InitialOutput=0
  wires:
  Sum4/1 -> Out1/1
  Memory1/1 -> Sum4/2
  Clock/1 -> Memory1/1, Sum4/1

== system lib_controls/<vc> insight/pre-TX parallel gearbox control/shifting1/time since last shift ==
  in_1 : Inport
  just shifted : Subsystem
      mask Display: disp('just\nshifted')
  timer : Subsystem
      mask Display: disp('timer')
  out_1 : Outport  InitialOutput=0
  wires:
  timer/1(time) -> out_1/1
  just shifted/1(out_1) -> timer/1(trigger)
  in_1/1 -> just shifted/1(in_1)

== system lib_controls/<vc> insight/pre-TX parallel gearbox control/upshift  command/load fraction ==
  In1 : Inport
  S-Function : S-Function  FunctionName=sfun_gearbox  Parameters=load, spd  EnableBusSupport=off
  Out1 : Outport  InitialOutput=0
  wires:
  S-Function/1 -> Out1/1
  In1/1 -> S-Function/1

== system lib_controls/<vc> par/parallel clutch control/gearbox speed estimator/Block NOTES ==
  note: The requested engine speed is replaced by an estimate of the
      | engine's previous speed whenever the vehicle missed the trace
      |  by more than 1 mph on the last time step.

== system lib_controls/<vc> par/parallel clutch control/gearbox speed estimator/dt ==
  Clock : Clock
  Memory1 : Memory  X0=-1
  Sum4 : Sum  Inputs=+-  SaturateOnIntegerOverflow=on  InputSameDT=on  OutDataTypeStr=Inherit: Same as first input
  Out1 : Outport  InitialOutput=0
  wires:
  Clock/1 -> Sum4/1, Memory1/1
  Memory1/1 -> Sum4/2
  Sum4/1 -> Out1/1

== system lib_controls/<vc> par/pre-TX parallel gearbox control/allow upshift?/Block NOTES1 ==
  note: This block prevents an upshift if it the engine is not on and
      | the upshift would make the motor power low enough that it
      | could not provide the required input power.  However, an upshift
      | is allowed if to stay in the current gear would put the motor
      | beyond 95% of its maximum speed.
      |
      | This block is to be used in pretransmission parallel hybrids
      | (where the engine and motor torques are combined on the
      | engine side of the transmission) ONLY.

== system lib_controls/<vc> par/pre-TX parallel gearbox control/downshift  command/load fraction ==
  In1 : Inport
  S-Function : S-Function  FunctionName=sfun_gearbox  Parameters=load, spd  EnableBusSupport=off
  Out1 : Outport  InitialOutput=0
  wires:
  In1/1 -> S-Function/1
  S-Function/1 -> Out1/1

== system lib_controls/<vc> par/pre-TX parallel gearbox control/gearbox speed estimator/Block NOTES ==
  note: The requested engine speed is replaced by an estimate of the
      | engine's previous speed whenever the vehicle missed the trace
      |  by more than 1 mph on the last time step.

== system lib_controls/<vc> par/pre-TX parallel gearbox control/gearbox speed estimator/dt ==
  Clock : Clock
  Memory1 : Memory  X0=-1
  Sum4 : Sum  Inputs=+-  SaturateOnIntegerOverflow=on  InputSameDT=on  OutDataTypeStr=Inherit: Same as first input
  Out1 : Outport  InitialOutput=0
  wires:
  Clock/1 -> Sum4/1, Memory1/1
  Memory1/1 -> Sum4/2
  Sum4/1 -> Out1/1

== system lib_controls/<vc> par/pre-TX parallel gearbox control/shifting1/time since last shift ==
  in_1 : Inport
  just shifted : Subsystem
      mask Display: disp('just\nshifted')
  timer : Subsystem
      mask Display: disp('timer')
  out_1 : Outport  InitialOutput=0
  wires:
  in_1/1 -> just shifted/1(in_1)
  just shifted/1(out_1) -> timer/1(trigger)
  timer/1(time) -> out_1/1

== system lib_controls/<vc> par/pre-TX parallel gearbox control/upshift  command/load fraction ==
  In1 : Inport
  S-Function : S-Function  FunctionName=sfun_gearbox  Parameters=load, spd  EnableBusSupport=off
  Out1 : Outport  InitialOutput=0
  wires:
  In1/1 -> S-Function/1
  S-Function/1 -> Out1/1

== system lib_controls/<vc> par Adaptive/engine on (Adaptive)/speed command/Block NOTES ==
  note: This engine control block determines whether the engine is on, which it is when
      | [(the clutch is slipping or engaged OR idling is allowed) AND the ignition key is on]
      | OR
      | (the transmission is shifting AND the engine was on during the previous time step).
      | The second part involving shifting is to prevent the engine from shutting down
      | for 1 or 2 seconds during shifts.

== system lib_controls/<vc> par Adaptive/engine on (Adaptive)/speed command/setpoint ==
  clutch state : Inport
  v_ave_req : Inport  Port=2
  Constant4 : Constant
  Constant5 : Constant  Value=0
  Constant6 : Constant  Value=0
  Logical Operator10 : Logic  Inputs=3
  clutch disengaged : RelationalOperator  Operator===  InputSameDT=on
  moving next time : RelationalOperator  Operator=>  InputSameDT=on
  not moving : RelationalOperator  Operator===  InputSameDT=on
  repeated cycle:  speed required at end of NEXT second : Subsystem  mask(Repeating table){t=cyc_mph(:,1), y=cyc_mph(:,2), dt=1}
      mask prompts: t "Time values:"; y "Output values:"; dt "Look ahead how far (s):"
      mask help:
      | Repeating table.
      | Enter values of time and output for first cycle.
      mask init:
      | period = max(t);
      mask Help: Repeats cycle given in table. Time values should be monotonically increasing.
  output : Outport
  wires:
  Logical Operator10/1 -> output/1
  v_ave_req/1 -> not moving/1
  clutch state/1 -> clutch disengaged/1
  Constant4/1 -> clutch disengaged/2
  Constant5/1 -> not moving/2
  repeated cycle:  speed required at end of NEXT second/1(out_1) -> moving next time/1
  Constant6/1 -> moving next time/2
  clutch disengaged/1 -> Logical Operator10/1
  not moving/1 -> Logical Operator10/2
  moving next time/1 -> Logical Operator10/3

== system lib_controls/<vc> par Adaptive/parallel clutch control/gearbox speed estimator/Block NOTES ==
  note: The requested engine speed is replaced by an estimate of the
      | engine's previous speed whenever the vehicle missed the trace
      |  by more than 1 mph on the last time step.

== system lib_controls/<vc> par Adaptive/parallel clutch control/gearbox speed estimator/dt ==
  Clock : Clock
  Memory1 : Memory  X0=-1
  Sum4 : Sum  Inputs=+-  SaturateOnIntegerOverflow=on  InputSameDT=on  OutDataTypeStr=Inherit: Same as first input
  Out1 : Outport  InitialOutput=0
  wires:
  Clock/1 -> Sum4/1, Memory1/1
  Memory1/1 -> Sum4/2
  Sum4/1 -> Out1/1

== system lib_controls/<vc> par Adaptive/pre-TX parallel gearbox control/allow upshift?/Block NOTES1 ==
  note: This block prevents an upshift if it the engine is not on and
      | the upshift would make the motor power low enough that it
      | could not provide the required input power.  However, an upshift
      | is allowed if to stay in the current gear would put the motor
      | beyond 95% of its maximum speed.
      |
      | This block is to be used in pretransmission parallel hybrids
      | (where the engine and motor torques are combined on the
      | engine side of the transmission) ONLY.

== system lib_controls/<vc> par Adaptive/pre-TX parallel gearbox control/downshift  command/load fraction ==
  In1 : Inport
  S-Function : S-Function  FunctionName=sfun_gearbox  Parameters=load, spd  EnableBusSupport=off
  Out1 : Outport  InitialOutput=0
  wires:
  In1/1 -> S-Function/1
  S-Function/1 -> Out1/1

== system lib_controls/<vc> par Adaptive/pre-TX parallel gearbox control/gearbox speed estimator/Block NOTES ==
  note: The requested engine speed is replaced by an estimate of the
      | engine's previous speed whenever the vehicle missed the trace
      |  by more than 1 mph on the last time step.

== system lib_controls/<vc> par Adaptive/pre-TX parallel gearbox control/gearbox speed estimator/dt ==
  Clock : Clock
  Memory1 : Memory  X0=-1
  Sum4 : Sum  Inputs=+-  SaturateOnIntegerOverflow=on  InputSameDT=on  OutDataTypeStr=Inherit: Same as first input
  Out1 : Outport  InitialOutput=0
  wires:
  Clock/1 -> Sum4/1, Memory1/1
  Memory1/1 -> Sum4/2
  Sum4/1 -> Out1/1

== system lib_controls/<vc> par Adaptive/pre-TX parallel gearbox control/shifting1/time since last shift ==
  in_1 : Inport
  just shifted : Subsystem
      mask Display: disp('just\nshifted')
  timer : Subsystem
      mask Display: disp('timer')
  out_1 : Outport  InitialOutput=0
  wires:
  in_1/1 -> just shifted/1(in_1)
  just shifted/1(out_1) -> timer/1(trigger)
  timer/1(time) -> out_1/1

== system lib_controls/<vc> par Adaptive/pre-TX parallel gearbox control/upshift  command/load fraction ==
  In1 : Inport
  S-Function : S-Function  FunctionName=sfun_gearbox  Parameters=load, spd  EnableBusSupport=off
  Out1 : Outport  InitialOutput=0
  wires:
  In1/1 -> S-Function/1
  S-Function/1 -> Out1/1

== system lib_controls/<vc> par auto/gearbox control for use w/ AT/downshift  command/load fraction ==
  In1 : Inport
  S-Function : S-Function  FunctionName=sfun_gearbox  Parameters=load, spd  EnableBusSupport=off
  Out1 : Outport  InitialOutput=0
  wires:
  S-Function/1 -> Out1/1
  In1/1 -> S-Function/1

== system lib_controls/<vc> par auto/gearbox control for use w/ AT/downshift  command1/load fraction ==
  In1 : Inport
  S-Function : S-Function  FunctionName=sfun_gearbox  Parameters=load, spd  EnableBusSupport=off
  Out1 : Outport  InitialOutput=0
  wires:
  In1/1 -> S-Function/1
  S-Function/1 -> Out1/1

== system lib_controls/<vc> par auto/gearbox control for use w/ AT/est. engine trq and spd/Block NOTES ==
  note: Estimate engine torque and speed associated with the previous gear, assuming that
      | the gearbox efficiency is constant.

== system lib_controls/<vc> par auto/gearbox control for use w/ AT/est. engine trq and spd/K_adv ==
  "Req'd output trq and spd (Nm), (rad/s)" : Inport
  K_adv=wout/(Tout)^0.5 : Fcn  Expr=u[2]/u[1]^0.5
  Saturation : Saturate  UpperLimit=max(htc_k_adv)  LowerLimit=min(htc_k_adv)
  Saturation2 : Saturate  UpperLimit=inf  LowerLimit=eps
  K_adv : Outport
  wires:
  "Req'd output trq and spd (Nm), (rad/s)"/1 -> Saturation2/1
  Saturation2/1 -> K_adv=wout/(Tout)^0.5/1
  K_adv=wout/(Tout)^0.5/1 -> Saturation/1
  Saturation/1 -> K_adv/1

== system lib_controls/<vc> par auto/gearbox control for use w/ AT/est. engine trq and spd assuming lockup/Block NOTES ==
  note: Estimate engine torque and speed associated with the current gear, assuming that
      | the gearbox efficiency is constant.
